simulink library "SMDFR_lib"  (R2024b)
settings: Solver=VariableStepAuto  StartTime=0.0  StopTime=10.0  RelTol=1e-3
undefined symbols (not defined in the file or in its folder): A_cucl, A_cucl2, A_cuocl, A_d, A_fw, A_h, A_h2, A_h20, A_hcl, A_o, A_wc, alfa_c, alfa_f, beta, beta_i, C_cucl, C_cuocl, C_dst, C_h20, C_hcl, C_hst, C_i0, C_o, c_pc, c_pf, c_pw, Ce_i0, d_dst, d_hst, DiscIntNeverNeededParam, E_d, E_e, E_h, E_hte, eta, G_cucl, G_cucl2, G_cuocl, G_h2, G_h20, G_h20i, G_h20o, G_hcl, G_o, h_dpo, h_fw, h_hpo, h_in, h_out, h_wc, k_d, K_d, k_e, k_h, K_h, k_hte, L, Lambda, lambda_c, lambda_e ... (+38)
libraries: simulink x1
settings Model: Creator=ste08  LastModifiedBy=stefanomarchetti
settings RTWCC: GPUComputeCapability=3.5

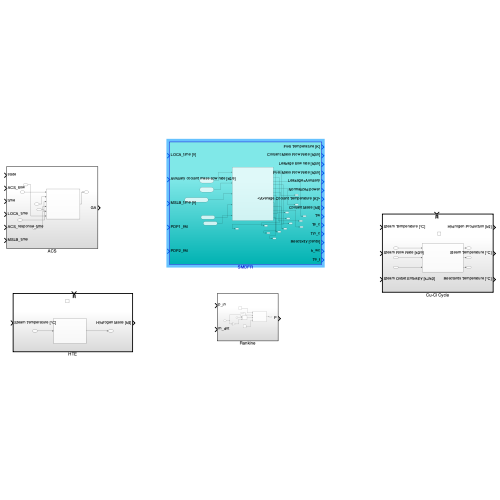
[thumbnail: Simulink's stored preview of the top-level diagram]
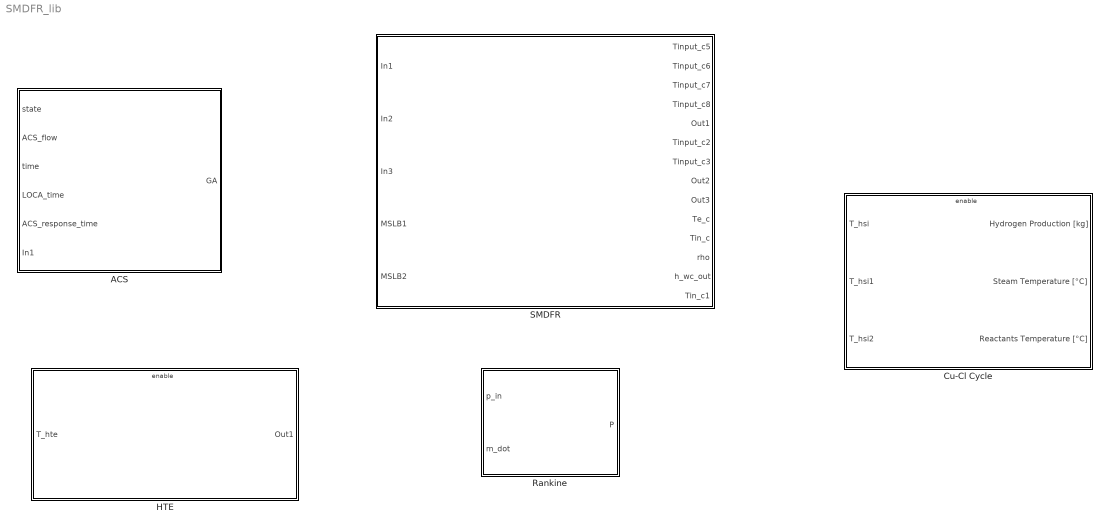
== system SMDFR_lib ==
  ACS : Subsystem
  Cu-Cl Cycle : Subsystem
  HTE : Subsystem
  Rankine : Subsystem
  SMDFR : Subsystem

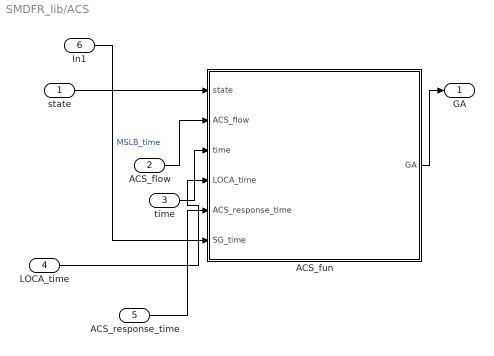
== system SMDFR_lib/ACS ==
  state : Inport
  ACS_flow : Inport  Port=2
  time : Inport  Port=3
  LOCA_time : Inport  Port=4
  ACS_response_time : Inport  Port=5
  In1 : Inport  Port=6
  ACS_fun : MATLAB Function  TreatAsAtomicUnit=on
  GA : Outport
  wires:
  ACS_flow/1 -> ACS_fun/2(ACS_flow)
  state/1 -> ACS_fun/1(state)
  ACS_fun/1(GA) -> GA/1
  time/1 -> ACS_fun/3(time)
  LOCA_time/1 -> ACS_fun/4(LOCA_time)
  ACS_response_time/1 -> ACS_fun/5(ACS_response_time)
  In1/1 -> ACS_fun/6(SG_time)  "MSLB_time"

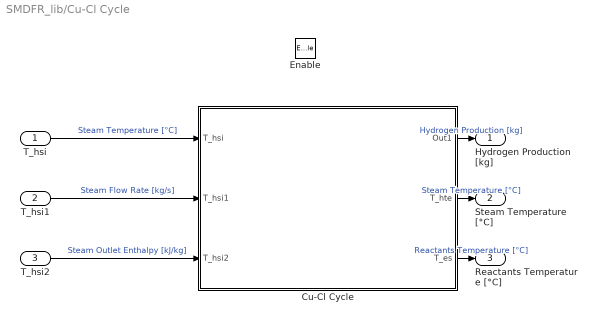
== system SMDFR_lib/Cu-Cl Cycle ==
  T_hsi : Inport
  T_hsi1 : Inport  Port=2
  T_hsi2 : Inport  Port=3
  Enable : EnablePort  StatesWhenEnabling=reset
  Cu-Cl Cycle : Subsystem
  Hydrogen Production [kg] : Outport
  Steam Temperature [°C] : Outport  Port=2
  Reactants Temperature [°C] : Outport  Port=3
  wires:
  Cu-Cl Cycle/1(Out1) -> Hydrogen Production [kg]/1  "Hydrogen Production [kg]"
  T_hsi/1 -> Cu-Cl Cycle/1(T_hsi)  "Steam Temperature [°C]"
  T_hsi1/1 -> Cu-Cl Cycle/2(T_hsi1)  "Steam Flow Rate [kg/s]"
  T_hsi2/1 -> Cu-Cl Cycle/3(T_hsi2)  "Steam Outlet Enthalpy [kJ/kg]"
  Cu-Cl Cycle/3(T_es) -> Reactants Temperature [°C]/1  "Reactants Temperature [°C]"
  Cu-Cl Cycle/2(T_hte) -> Steam Temperature [°C]/1  "Steam Temperature [°C]"

== system SMDFR_lib/HTE ==
  T_hte : Inport
  Enable : EnablePort  StatesWhenEnabling=reset
  HTE : Subsystem
  Out1 : Outport
  wires:
  HTE/1(Out2) -> Out1/1  "Hydrogen Mass [kg]"
  T_hte/1 -> HTE/1(T_hte)  "Steam Temperature [°C]"

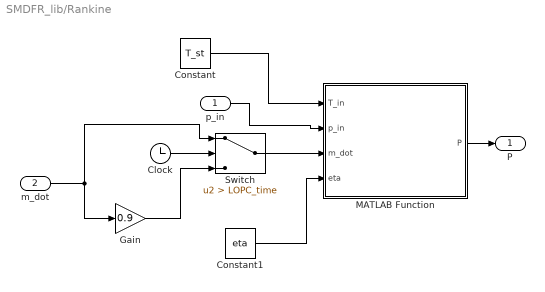
== system SMDFR_lib/Rankine ==
  p_in : Inport
  m_dot : Inport  Port=2
  Clock : Clock
  Constant : Constant  Value=T_st
  Constant1 : Constant  Value=eta
  Gain : Gain  Gain=0.9
  MATLAB Function : MATLAB Function  TreatAsAtomicUnit=on
  Switch : Switch  Criteria=u2 > Threshold  Threshold=LOPC_time  SaturateOnIntegerOverflow=off  InputSameDT=off
  P : Outport
  wires:
  p_in/1 -> MATLAB Function/2(p_in)
  m_dot/1 -> Switch/1, Gain/1
  MATLAB Function/1(P) -> P/1
  Constant/1 -> MATLAB Function/1(T_in)
  Constant1/1 -> MATLAB Function/4(eta)
  Clock/1 -> Switch/2
  Switch/1 -> MATLAB Function/3(m_dot)
  Gain/1 -> Switch/3

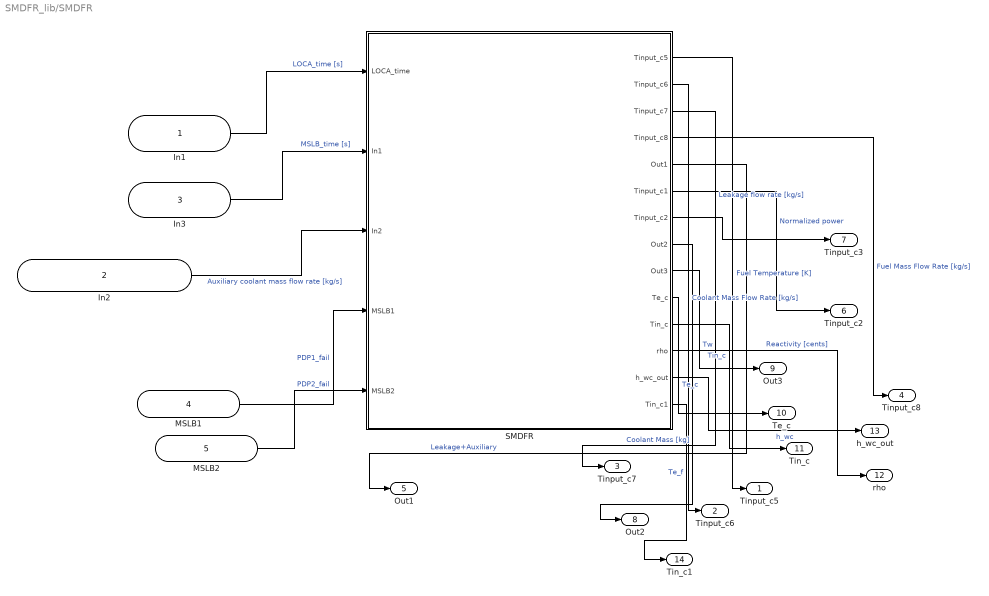
== system SMDFR_lib/SMDFR ==
  In1 : Inport
  In2 : Inport  Port=2
  In3 : Inport  Port=3
  MSLB1 : Inport  Port=4
  MSLB2 : Inport  Port=5
  SMDFR : Subsystem
  Tinput_c5 : Outport
  Tinput_c6 : Outport  Port=2
  Tinput_c7 : Outport  Port=3
  Tinput_c8 : Outport  Port=4
  Out1 : Outport  Port=5
  Tinput_c2 : Outport  Port=6
  Tinput_c3 : Outport  Port=7
  Out2 : Outport  Port=8
  Out3 : Outport  Port=9
  Te_c : Outport  Port=10
  Tin_c : Outport  Port=11
  rho : Outport  Port=12
  h_wc_out : Outport  Port=13
  Tin_c1 : Outport  Port=14
  wires:
  In1/1 -> SMDFR/1(LOCA_time)  "LOCA_time [s]"
  SMDFR/1(Tinput_c5) -> Tinput_c5/1  "Fuel Temperature [K]"
  SMDFR/2(Tinput_c6) -> Tinput_c6/1  "Coolant Mass Flow Rate [kg/s]"
  In2/1 -> SMDFR/3(In2)  "Auxiliary coolant mass flow rate [kg/s]"
  SMDFR/3(Tinput_c7) -> Tinput_c7/1  "Leakage flow rate [kg/s]"
  SMDFR/4(Tinput_c8) -> Tinput_c8/1  "Fuel Mass Flow Rate [kg/s]"
  SMDFR/5(Out1) -> Out1/1  "Leakage+Auxiliary"
  SMDFR/6(Tinput_c1) -> Tinput_c2/1  "Normalized power"
  SMDFR/7(Tinput_c2) -> Tinput_c3/1
  SMDFR/8(Out2) -> Out2/1  "Coolant Mass [kg]"
  SMDFR/9(Out3) -> Out3/1  "Tw"
  SMDFR/10(Te_c) -> Te_c/1  "Te_c"
  SMDFR/11(Tin_c) -> Tin_c/1  "Tin_c"
  SMDFR/12(rho) -> rho/1  "Reactivity [cents]"
  SMDFR/13(h_wc_out) -> h_wc_out/1  "h_wc"
  SMDFR/14(Tin_c1) -> Tin_c1/1  "Te_f"
  In3/1 -> SMDFR/2(In1)  "MSLB_time [s]"
  MSLB1/1 -> SMDFR/4(MSLB1)  "PDP1_fail"
  MSLB2/1 -> SMDFR/5(MSLB2)  "PDP2_fail"

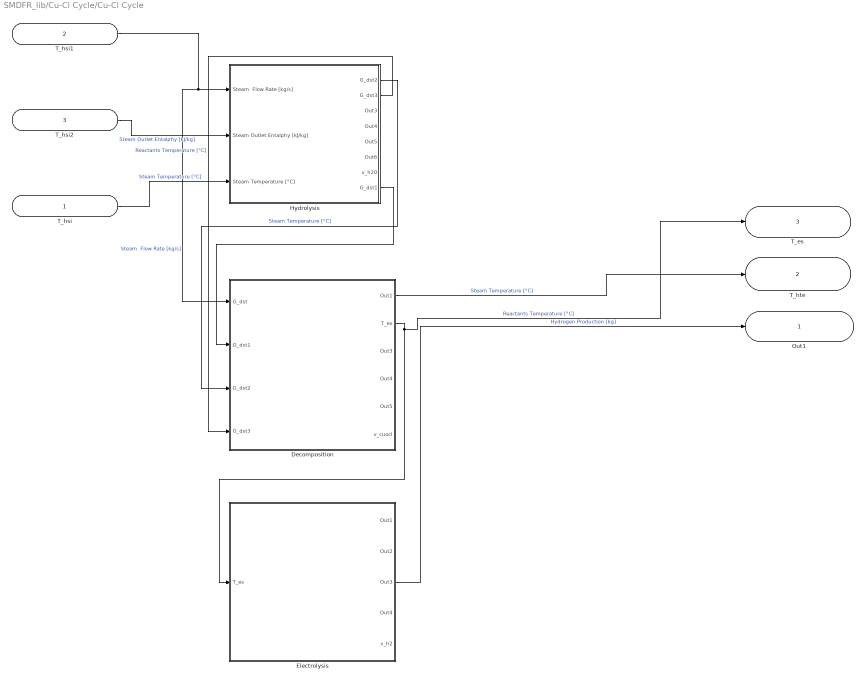
== system SMDFR_lib/Cu-Cl Cycle/Cu-Cl Cycle ==
  T_hsi : Inport
  T_hsi1 : Inport  Port=2
  T_hsi2 : Inport  Port=3
  Decomposition : Subsystem
  Electrolysis : Subsystem
  Hydrolysis : Subsystem
  Out1 : Outport
  T_hte : Outport  Port=2
  T_es : Outport  Port=3
  wires:
  T_hsi2/1 -> Hydrolysis/2(Steam Outlet Entalphy [kJ/kg])  "Steam Outlet Entalphy [kJ/kg]"
  T_hsi/1 -> Hydrolysis/3(Steam Temperature [°C])  "Steam Temperature [°C]"
  Hydrolysis/1(G_dst2) -> Decomposition/3(G_dst2)  "Steam Temperature [°C]"
  Hydrolysis/2(G_dst3) -> Decomposition/4(G_dst3)  "Reactants Temperature [°C]"
  Hydrolysis/8(G_dst1) -> Decomposition/2(G_dst1)
  Decomposition/1(Out1) -> T_hte/1  "Steam Temperature [°C]"
  Decomposition/2(T_es) -> Electrolysis/1(T_es), T_es/1  "Reactants Temperature [°C]"
  Electrolysis/3(Out3) -> Out1/1  "Hydrogen Production [kg]"
  T_hsi1/1 -> Decomposition/1(G_dst), Hydrolysis/1(Steam  Flow Rate [kg/s])  "Steam  Flow Rate [kg/s]"

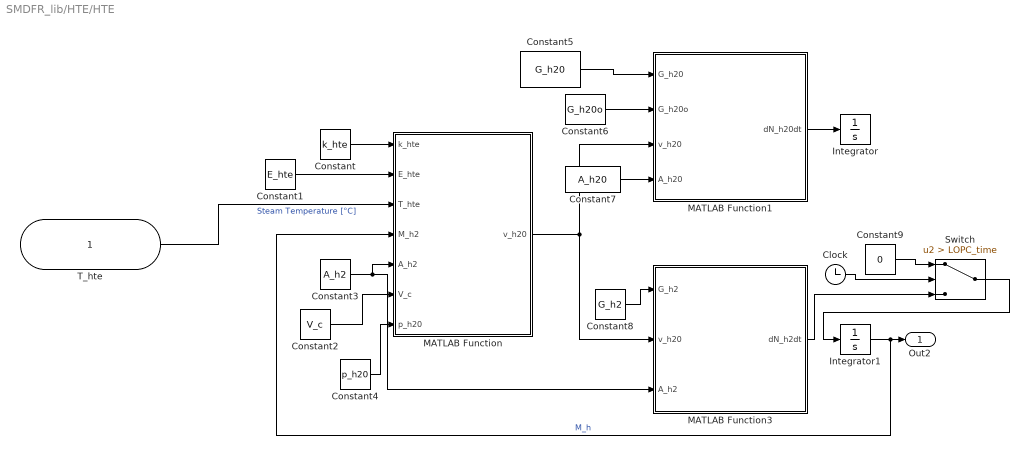
== system SMDFR_lib/HTE/HTE ==
  T_hte : Inport
  Clock : Clock
  Constant : Constant  Value=k_hte
  Constant1 : Constant  Value=E_hte
  Constant2 : Constant  Value=V_c
  Constant3 : Constant  Value=A_h2
  Constant4 : Constant  Value=p_h20
  Constant5 : Constant  Value=G_h20
  Constant6 : Constant  Value=G_h20o
  Constant7 : Constant  Value=A_h20
  Constant8 : Constant  Value=G_h2
  Constant9 : Constant  Value=0
  Integrator : Integrator  InitialCondition=100
  Integrator1 : Integrator  InitialCondition=100
  MATLAB Function : MATLAB Function  TreatAsAtomicUnit=on
  MATLAB Function1 : MATLAB Function  TreatAsAtomicUnit=on
  MATLAB Function3 : MATLAB Function  TreatAsAtomicUnit=on
  Switch : Switch  Criteria=u2 > Threshold  Threshold=LOPC_time  SaturateOnIntegerOverflow=off  InputSameDT=off
  Out2 : Outport
  wires:
  T_hte/1 -> MATLAB Function/3(T_hte)  "Steam Temperature [°C]"
  MATLAB Function/1(v_h20) -> MATLAB Function3/2(v_h20), MATLAB Function1/3(v_h20)
  Constant/1 -> MATLAB Function/1(k_hte)
  Constant1/1 -> MATLAB Function/2(E_hte)
  Constant3/1 -> MATLAB Function3/3(A_h2), MATLAB Function/5(A_h2)
  Constant2/1 -> MATLAB Function/6(V_c)
  Constant4/1 -> MATLAB Function/7(p_h20)
  Constant5/1 -> MATLAB Function1/1(G_h20)
  Constant6/1 -> MATLAB Function1/2(G_h20o)
  Constant7/1 -> MATLAB Function1/4(A_h20)
  Constant8/1 -> MATLAB Function3/1(G_h2)
  MATLAB Function1/1(dN_h20dt) -> Integrator/1
  Switch/1 -> Integrator1/1
  Integrator1/1 -> MATLAB Function/4(M_h2), Out2/1  "M_h"
  MATLAB Function3/1(dN_h2dt) -> Switch/3
  Constant9/1 -> Switch/1
  Clock/1 -> Switch/2

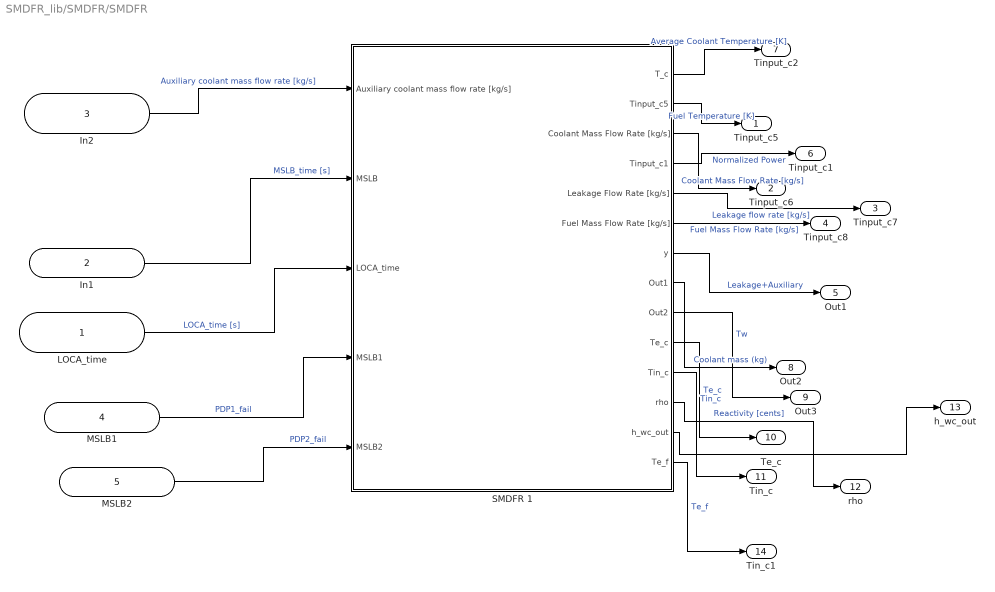
== system SMDFR_lib/SMDFR/SMDFR ==
  LOCA_time : Inport
  In1 : Inport  Port=2
  In2 : Inport  Port=3
  MSLB1 : Inport  Port=4
  MSLB2 : Inport  Port=5
  SMDFR 1 : Subsystem
  Tinput_c5 : Outport
  Tinput_c6 : Outport  Port=2
  Tinput_c7 : Outport  Port=3
  Tinput_c8 : Outport  Port=4
  Out1 : Outport  Port=5
  Tinput_c1 : Outport  Port=6
  Tinput_c2 : Outport  Port=7
  Out2 : Outport  Port=8
  Out3 : Outport  Port=9
  Te_c : Outport  Port=10
  Tin_c : Outport  Port=11
  rho : Outport  Port=12
  h_wc_out : Outport  Port=13
  Tin_c1 : Outport  Port=14
  wires:
  SMDFR 1/3(Coolant Mass Flow Rate [kg/s]) -> Tinput_c6/1  "Coolant Mass Flow Rate [kg/s]"
  SMDFR 1/2(Tinput_c5) -> Tinput_c5/1  "Fuel Temperature [K]"
  In2/1 -> SMDFR 1/1(Auxiliary coolant mass flow rate [kg/s])  "Auxiliary coolant mass flow rate [kg/s]"
  SMDFR 1/5(Leakage Flow Rate [kg/s]) -> Tinput_c7/1  "Leakage flow rate [kg/s]"
  SMDFR 1/6(Fuel Mass Flow Rate [kg/s]) -> Tinput_c8/1  "Fuel Mass Flow Rate [kg/s]"
  LOCA_time/1 -> SMDFR 1/3(LOCA_time)  "LOCA_time [s]"
  SMDFR 1/7(y) -> Out1/1  "Leakage+Auxiliary"
  SMDFR 1/4(Tinput_c1) -> Tinput_c1/1  "Normalized Power"
  SMDFR 1/1(T_c) -> Tinput_c2/1  "Average Coolant Temperature [K]"
  SMDFR 1/8(Out1) -> Out2/1  "Coolant mass (kg)"
  SMDFR 1/9(Out2) -> Out3/1  "Tw"
  SMDFR 1/10(Te_c) -> Te_c/1  "Te_c"
  SMDFR 1/11(Tin_c) -> Tin_c/1  "Tin_c"
  SMDFR 1/12(rho) -> rho/1  "Reactivity [cents]"
  SMDFR 1/13(h_wc_out) -> h_wc_out/1
  SMDFR 1/14(Te_f) -> Tin_c1/1  "Te_f"
  In1/1 -> SMDFR 1/2(MSLB)  "MSLB_time [s]"
  MSLB1/1 -> SMDFR 1/4(MSLB1)  "PDP1_fail"
  MSLB2/1 -> SMDFR 1/5(MSLB2)  "PDP2_fail"

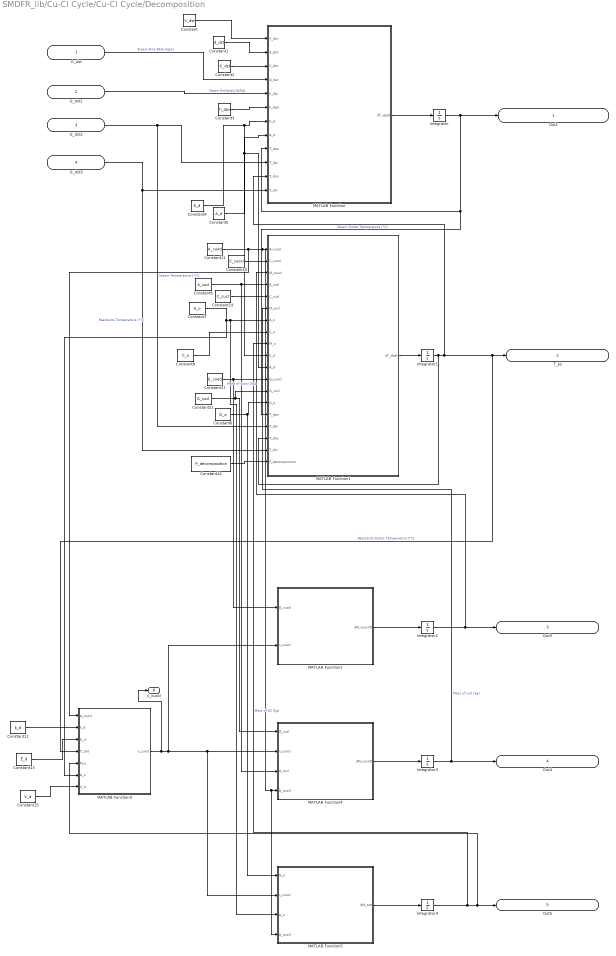
== system SMDFR_lib/Cu-Cl Cycle/Cu-Cl Cycle/Decomposition ==
  G_dst : Inport
  G_dst1 : Inport  Port=2
  G_dst2 : Inport  Port=3
  G_dst3 : Inport  Port=4
  Constant : Constant  Value=V_dst
  Constant1 : Constant  Value=d_dst
  Constant10 : Constant  Value=C_cuocl
  Constant11 : Constant  Value=A_cuocl
  Constant12 : Constant  Value=k_d
  Constant13 : Constant  Value=E_d
  Constant14 : Constant  Value=P_decomposition
  Constant15 : Constant  Value=V_d
  Constant17 : Constant  Value=G_cuocl
  Constant19 : Constant  Value=C_cucl
  Constant2 : Constant  Value=C_dst
  Constant21 : Constant  Value=G_cucl
  Constant3 : Constant  Value=h_dpo
  Constant4 : Constant  Value=K_d
  Constant5 : Constant  Value=A_d
  Constant6 : Constant  Value=G_o
  Constant7 : Constant  Value=A_o
  Constant8 : Constant  Value=C_o
  Constant9 : Constant  Value=A_cucl
  Integrator : Integrator  InitialCondition=1000
  Integrator{1..4} (4 alike) : Integrator  InitialCondition=100
  MATLAB Function : MATLAB Function  TreatAsAtomicUnit=on
  MATLAB Function1 : MATLAB Function  TreatAsAtomicUnit=on
  MATLAB Function2 : MATLAB Function  TreatAsAtomicUnit=on
  MATLAB Function3 : MATLAB Function  TreatAsAtomicUnit=on
  MATLAB Function4 : MATLAB Function  TreatAsAtomicUnit=on
  MATLAB Function5 : MATLAB Function  TreatAsAtomicUnit=on
  Out1 : Outport
  T_es : Outport  Port=2
  Out3 : Outport  Port=3
  Out4 : Outport  Port=4
  Out5 : Outport  Port=5
  v_cuocl : Outport  Port=6
  wires:
  MATLAB Function/1(dT_dpdt) -> Integrator/1
  G_dst/1 -> MATLAB Function/4(G_dst)  "Steam Flow Rate [kg/s]"
  G_dst1/1 -> MATLAB Function/5(h_dpi)  "Steam Enthalpy [kJ/kg]"
  G_dst2/1 -> MATLAB Function1/16(T_dpi), MATLAB Function/10(T_dpi)  "Steam Temperature [°C]"
  Constant/1 -> MATLAB Function/1(V_dst)
  Constant1/1 -> MATLAB Function/2(d_dst)
  Constant2/1 -> MATLAB Function/3(C_dst)
  Constant3/1 -> MATLAB Function/6(h_dpo)
  Constant4/1 -> MATLAB Function/7(K_d), MATLAB Function1/10(K_d)
  Constant5/1 -> MATLAB Function/8(A_d), MATLAB Function1/11(A_d)
  G_dst3/1 -> MATLAB Function1/18(T_dsi), MATLAB Function/12(T_dsi)  "Reactants Temperature [°C]"
  MATLAB Function1/1(dT_dsdt) -> Integrator1/1
  Integrator/1 -> MATLAB Function1/15(T_dpo), MATLAB Function/9(T_dpo), Out1/1  "Steam Outlet Temperature [°C]"
  Integrator1/1 -> MATLAB Function1/17(T_dso), MATLAB Function/11(T_dso), MATLAB Function3/4(T_dso), T_es/1  "Reactants Outlet Temperature [°C]"
  Constant11/1 -> MATLAB Function5/4(A_cuocl), MATLAB Function4/4(A_cuocl), MATLAB Function1/1(A_cuocl), MATLAB Function3/1(A_cuocl)
  Constant9/1 -> MATLAB Function4/3(A_cucl), MATLAB Function1/4(A_cucl)
  Constant21/1 -> MATLAB Function4/1(G_cucl), MATLAB Function1/13(G_cucl)
  Constant17/1 -> MATLAB Function2/1(G_cuocl), MATLAB Function1/12(G_cuocl)
  Constant6/1 -> MATLAB Function5/1(G_o), MATLAB Function1/14(G_o)
  Constant7/1 -> MATLAB Function3/6(A_o), MATLAB Function5/3(A_o), MATLAB Function1/7(A_o)
  Constant8/1 -> MATLAB Function1/8(C_o)
  Constant10/1 -> MATLAB Function1/2(C_cuocl)
  Constant19/1 -> MATLAB Function1/5(C_cucl)
  Constant14/1 -> MATLAB Function1/19(P_decomposition)
  MATLAB Function2/1(dM_cuocldt) -> Integrator2/1
  Integrator2/1 -> MATLAB Function1/3(M_cuocl), Out3/1  "Mass of cuocl [kg]"
  MATLAB Function3/1(v_cuocl) -> v_cuocl/1, MATLAB Function2/2(v_cuocl), MATLAB Function5/2(v_cuocl), MATLAB Function4/2(v_cuocl)
  MATLAB Function4/1(dM_cucldt) -> Integrator3/1
  Integrator3/1 -> MATLAB Function1/6(M_cucl), Out4/1  "Mass of cucl [kg]"
  MATLAB Function5/1(dM_odt) -> Integrator4/1
  Integrator4/1 -> MATLAB Function1/9(M_o), MATLAB Function3/5(M_o), Out5/1  "Mass of O2 [kg]"
  Constant15/1 -> MATLAB Function3/7(V_d)
  Constant13/1 -> MATLAB Function3/3(E_d)
  Constant12/1 -> MATLAB Function3/2(k_d)

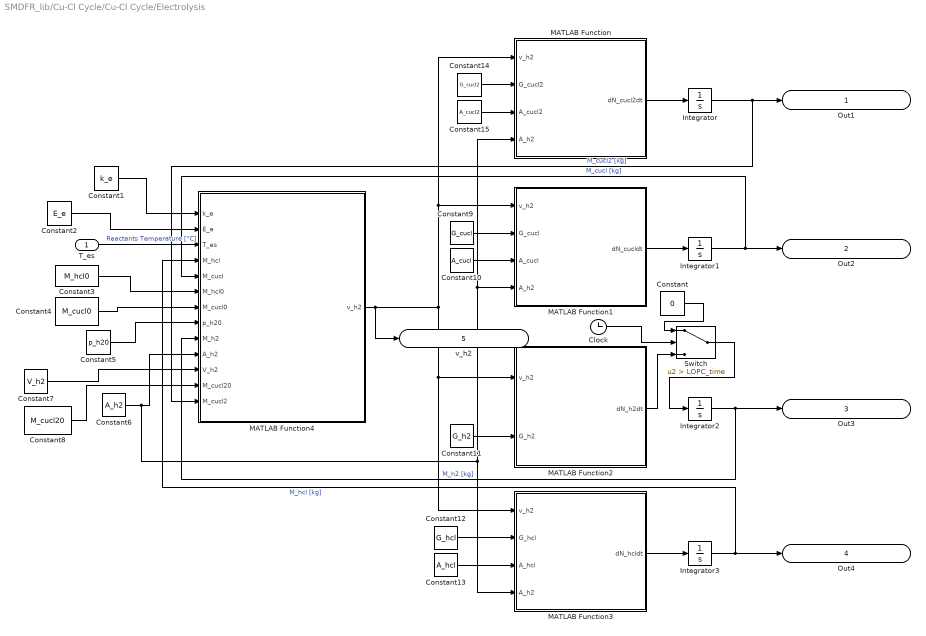
== system SMDFR_lib/Cu-Cl Cycle/Cu-Cl Cycle/Electrolysis ==
  T_es : Inport
  Clock : Clock
  Constant : Constant  Value=0
  Constant1 : Constant  Value=k_e
  Constant10 : Constant  Value=A_cucl
  Constant11 : Constant  Value=G_h2
  Constant12 : Constant  Value=G_hcl
  Constant13 : Constant  Value=A_hcl
  Constant14 : Constant  Value=G_cucl2
  Constant15 : Constant  Value=A_cucl2
  Constant2 : Constant  Value=E_e
  Constant3 : Constant  Value=M_hcl0
  Constant4 : Constant  Value=M_cucl0
  Constant5 : Constant  Value=p_h20
  Constant6 : Constant  Value=A_h2
  Constant7 : Constant  Value=V_h2
  Constant8 : Constant  Value=M_cucl20
  Constant9 : Constant  Value=G_cucl
  Integrator : Integrator  InitialCondition=M_cucl20
  Integrator1 : Integrator  InitialCondition=M_cucl0
  Integrator2 : Integrator  InitialCondition=M_h20
  Integrator3 : Integrator  InitialCondition=M_hcl0
  MATLAB Function : MATLAB Function  TreatAsAtomicUnit=on
  MATLAB Function1 : MATLAB Function  TreatAsAtomicUnit=on
  MATLAB Function2 : MATLAB Function  TreatAsAtomicUnit=on
  MATLAB Function3 : MATLAB Function  TreatAsAtomicUnit=on
  MATLAB Function4 : MATLAB Function  TreatAsAtomicUnit=on
  Switch : Switch  Criteria=u2 > Threshold  Threshold=LOPC_time  SaturateOnIntegerOverflow=off  InputSameDT=off
  Out1 : Outport
  Out2 : Outport  Port=2
  Out3 : Outport  Port=3
  Out4 : Outport  Port=4
  v_h2 : Outport  Port=5
  wires:
  MATLAB Function/1(dN_cucl2dt) -> Integrator/1
  MATLAB Function1/1(dN_cucldt) -> Integrator1/1
  Switch/1 -> Integrator2/1
  MATLAB Function3/1(dN_hcldt) -> Integrator3/1
  MATLAB Function4/1(v_h2) -> v_h2/1, MATLAB Function/1(v_h2), MATLAB Function1/1(v_h2), MATLAB Function3/1(v_h2), MATLAB Function2/1(v_h2)
  Integrator/1 -> MATLAB Function4/13(M_cucl2), Out1/1  "M_cucl2 [kg]"
  Integrator1/1 -> MATLAB Function4/5(M_cucl), Out2/1  "M_cucl [kg]"
  Integrator2/1 -> MATLAB Function4/9(M_h2), Out3/1  "M_h2 [kg]"
  Integrator3/1 -> MATLAB Function4/4(M_hcl), Out4/1  "M_hcl [kg]"
  T_es/1 -> MATLAB Function4/3(T_es)  "Reactants Temperature [°C]"
  Constant1/1 -> MATLAB Function4/1(k_e)
  Constant2/1 -> MATLAB Function4/2(E_e)
  Constant3/1 -> MATLAB Function4/6(M_hcl0)
  Constant4/1 -> MATLAB Function4/7(M_cucl0)
  Constant5/1 -> MATLAB Function4/8(p_h20)
  Constant6/1 -> MATLAB Function/4(A_h2), MATLAB Function1/4(A_h2), MATLAB Function3/4(A_h2), MATLAB Function4/10(A_h2)
  Constant7/1 -> MATLAB Function4/11(V_h2)
  Constant8/1 -> MATLAB Function4/12(M_cucl20)
  Constant9/1 -> MATLAB Function1/2(G_cucl)
  Constant10/1 -> MATLAB Function1/3(A_cucl)
  Constant11/1 -> MATLAB Function2/2(G_h2)
  Constant12/1 -> MATLAB Function3/2(G_hcl)
  Constant13/1 -> MATLAB Function3/3(A_hcl)
  Constant14/1 -> MATLAB Function/2(G_cucl2)
  Constant15/1 -> MATLAB Function/3(A_cucl2)
  MATLAB Function2/1(dN_h2dt) -> Switch/3
  Clock/1 -> Switch/2
  Constant/1 -> Switch/1

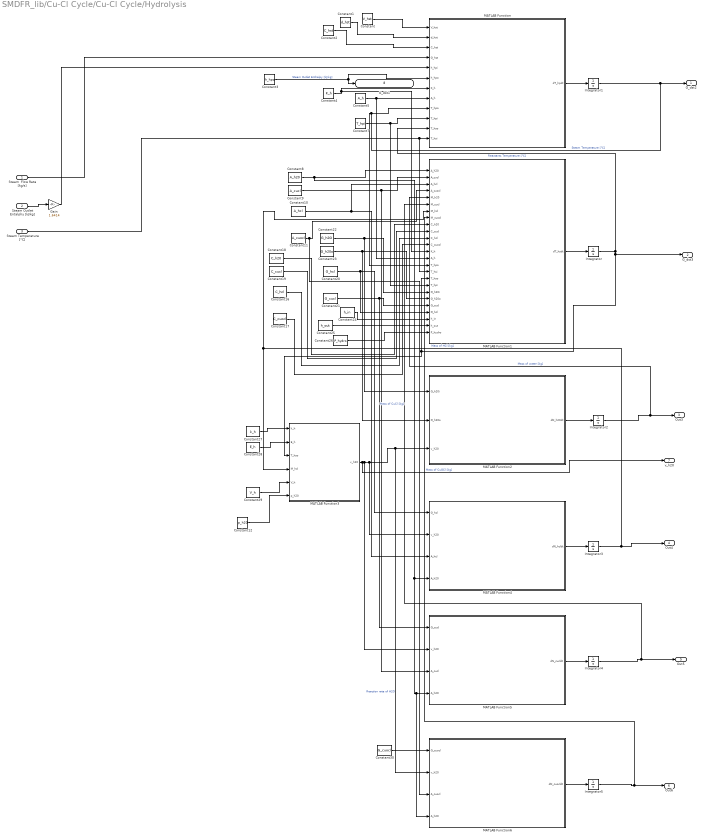
== system SMDFR_lib/Cu-Cl Cycle/Cu-Cl Cycle/Hydrolysis ==
  Steam  Flow Rate [kg/s] : Inport
  Steam Outlet Entalphy [kJ/kg] : Inport  Port=2
  Steam Temperature [°C] : Inport  Port=3
  Constant : Constant  Value=V_hst
  Constant1 : Constant  Value=d_hst
  Constant10 : Constant  Value=A_hcl
  Constant11 : Constant  Value=A_cuocl
  Constant12 : Constant  Value=p_h20
  Constant16 : Constant  Value=C_hcl
  Constant17 : Constant  Value=C_cuocl
  Constant18 : Constant  Value=C_h20
  Constant19 : Constant  Value=C_cucl
  Constant2 : Constant  Value=C_hst
  Constant20 : Constant  Value=G_hcl
  Constant21 : Constant  Value=G_cucl
  Constant22 : Constant  Value=G_h20i
  Constant23 : Constant  Value=G_h20o
  Constant24 : Constant  Value=h_in
  Constant25 : Constant  Value=h_out
  Constant26 : Constant  Value=P_hydro
  Constant27 : Constant  Value=k_h
  Constant28 : Constant  Value=E_h
  Constant29 : Constant  Value=V_h
  Constant3 : Constant  Value=h_hpo
  Constant30 : Constant  Value=G_cuocl
  Constant4 : Constant  Value=K_h
  Constant5 : Constant  Value=A_h
  Constant7 : Constant  Value=T_hpi
  Constant8 : Constant  Value=A_h20
  Constant9 : Constant  Value=A_cucl
  Gain : Gain  Gain=1.6414
  Integrator : Integrator  InitialCondition=T_hpi-50
  Integrator1 : Integrator  InitialCondition=T_st+100
  Integrator2 : Integrator  InitialCondition=200
  Integrator3 : Integrator  InitialCondition=50
  Integrator4 : Integrator  InitialCondition=200
  Integrator5 : Integrator  InitialCondition=50
  MATLAB Function : MATLAB Function  TreatAsAtomicUnit=on
  MATLAB Function1 : MATLAB Function  TreatAsAtomicUnit=on
  MATLAB Function2 : MATLAB Function  TreatAsAtomicUnit=on
  MATLAB Function3 : MATLAB Function  TreatAsAtomicUnit=on
  MATLAB Function4 : MATLAB Function  TreatAsAtomicUnit=on
  MATLAB Function5 : MATLAB Function  TreatAsAtomicUnit=on
  MATLAB Function6 : MATLAB Function  TreatAsAtomicUnit=on
  G_dst2 : Outport
  G_dst3 : Outport  Port=2
  Out3 : Outport  Port=3
  Out4 : Outport  Port=4
  Out5 : Outport  Port=5
  Out6 : Outport  Port=6
  v_h20 : Outport  Port=7
  G_dst1 : Outport  Port=8
  wires:
  Constant23/1 -> MATLAB Function2/2(G_h20o), MATLAB Function1/20(G_h20o)
  MATLAB Function3/1(v_h20) -> v_h20/1, MATLAB Function5/2(v_h20), MATLAB Function4/2(v_h20), MATLAB Function6/2(v_h20), MATLAB Function2/3(v_h20)  "Reaction rate of H2O"
  Constant8/1 -> MATLAB Function6/4(A_h20), MATLAB Function5/4(A_h20), MATLAB Function4/4(A_h20), MATLAB Function1/1(A_h20)
  Integrator2/1 -> MATLAB Function1/5(M_h20), Out3/1  "Mass of water [kg]"
  Constant26/1 -> MATLAB Function1/25(P_hydro)
  Constant/1 -> MATLAB Function/1(V_hst)
  Integrator4/1 -> MATLAB Function1/6(M_cucl), Out5/1  "Mass of CuCl [kg]"
  Constant27/1 -> MATLAB Function3/1(k_h)
  Integrator/1 -> G_dst3/1, MATLAB Function3/3(T_hso), MATLAB Function1/17(T_hso), MATLAB Function/11(T_hso)  "Reactants Temperature [°C]"
  Constant25/1 -> MATLAB Function1/24(h_out)
  Steam Temperature [°C]/1 -> MATLAB Function1/16(T_hsi), MATLAB Function/12(T_hsi)
  Constant28/1 -> MATLAB Function3/2(E_h)
  Constant24/1 -> MATLAB Function1/23(h_in)
  Constant3/1 -> G_dst1/1, MATLAB Function/6(h_hpo)  "Steam Outlet Enthalpy [kJ/kg]"
  Constant1/1 -> MATLAB Function/2(d_hst)
  Integrator1/1 -> MATLAB Function1/15(T_hpo), MATLAB Function/9(T_hpo), G_dst2/1  "Steam Temperature [°C]"
  Constant20/1 -> MATLAB Function4/1(G_hcl), MATLAB Function1/22(G_hcl)
  Constant7/1 -> MATLAB Function1/18(T_hpi), MATLAB Function/10(T_hpi)
  Constant2/1 -> MATLAB Function/3(C_hst)
  Gain/1 -> MATLAB Function/5(h_hpi)
  Constant22/1 -> MATLAB Function2/1(G_h20i), MATLAB Function1/19(G_h20i)
  Constant9/1 -> MATLAB Function5/3(A_cucl), MATLAB Function1/2(A_cucl)
  Constant21/1 -> MATLAB Function5/1(G_cucl), MATLAB Function1/21(G_cucl)
  Constant4/1 -> MATLAB Function1/13(K_h), MATLAB Function/7(K_h)
  Constant11/1 -> MATLAB Function6/3(A_cuocl), MATLAB Function1/4(A_cuocl)
  Constant19/1 -> MATLAB Function1/10(C_cucl)
  Integrator5/1 -> MATLAB Function1/8(M_cuocl), Out6/1  "Mass of CuOCl [kg]"
  MATLAB Function4/1(dN_hcldt) -> Integrator3/1
  Constant29/1 -> MATLAB Function3/5(V_h)
  Constant16/1 -> MATLAB Function1/11(C_hcl)
  MATLAB Function6/1(dN_cuocldt) -> Integrator5/1
  Constant17/1 -> MATLAB Function1/12(C_cuocl)
  Constant10/1 -> MATLAB Function4/3(A_hcl), MATLAB Function1/3(A_hcl)
  MATLAB Function5/1(dN_cucldt) -> Integrator4/1
  MATLAB Function/1(dT_hpdt) -> Integrator1/1
  Constant5/1 -> MATLAB Function1/14(A_h), MATLAB Function/8(A_h)
  Constant30/1 -> MATLAB Function6/1(G_cuocl)
  MATLAB Function1/1(dT_hsdt) -> Integrator/1
  Constant18/1 -> MATLAB Function1/9(C_h20)
  Integrator3/1 -> Out4/1, MATLAB Function1/7(M_hcl), MATLAB Function3/4(M_hcl)  "Mass of HCl [kg]"
  MATLAB Function2/1(dN_h20dt) -> Integrator2/1
  Steam  Flow Rate [kg/s]/1 -> MATLAB Function/4(G_hst)
  Constant12/1 -> MATLAB Function3/6(p_h20)
  Steam Outlet Entalphy [kJ/kg]/1 -> Gain/1

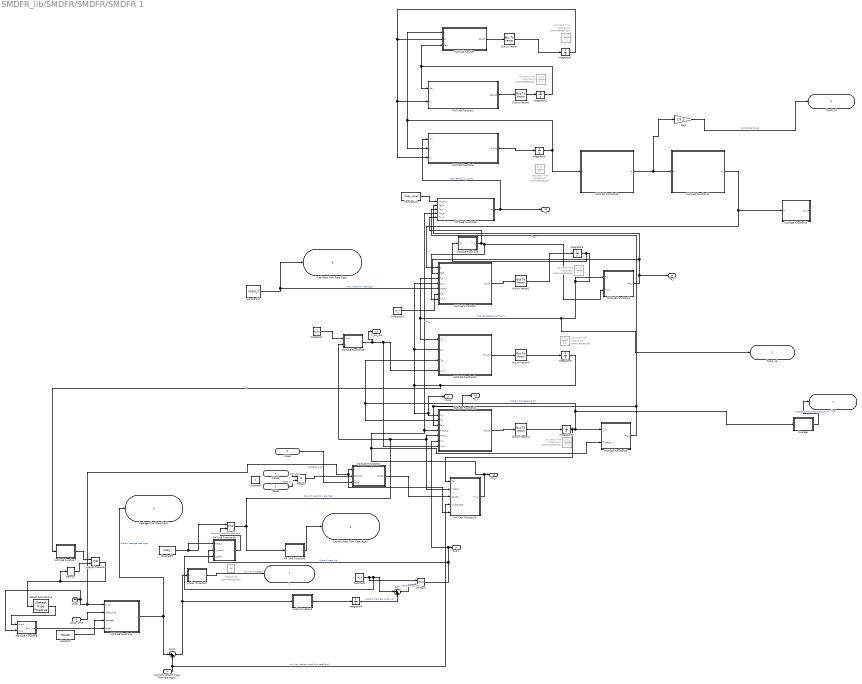
== system SMDFR_lib/SMDFR/SMDFR/SMDFR 1 ==
  Auxiliary coolant mass flow rate [kg/s] : Inport
  MSLB : Inport  Port=2
  LOCA_time : Inport  Port=3
  MSLB1 : Inport  Port=4
  MSLB2 : Inport  Port=5
  Average : MATLAB Function  TreatAsAtomicUnit=on
  Bus to Vector{,1..4} (5 alike) : BusToVector
  Clock : Clock
  Constant : Constant  Value=leakage
  Constant1 : Constant  Value=M_c
  Constant13 : Constant  Value=rhoex_value  SampleTime=-1
  Constant17 : Constant  Value=mdot_f  SampleTime=-1
  Constant2 : Constant  Value=h_wc
  Constant20 : Constant  Value=M_f  SampleTime=-1
  Constant3 : Constant
  Constant9 : Constant  Value=mdot_c  SampleTime=-1
  Detect Rise Positive : simulink/Logic and Bit Operations/Detect Rise Positive  vinit=0  OutDataTypeStr=boolean
  Discrete-Time Integrator : DiscreteIntegrator  Commented=on  InitialCondition=Tf_0  SampleTime=-1  ICPrevOutput=DiscIntNeverNeededParam  ICPrevScaledInput=DiscIntNeverNeededParam
  Discrete-Time Integrator2 : DiscreteIntegrator  Commented=on  InitialCondition=N_0  SampleTime=-1  ICPrevOutput=DiscIntNeverNeededParam  ICPrevScaledInput=DiscIntNeverNeededParam
  Discrete-Time Integrator3 : DiscreteIntegrator  Commented=on  InitialCondition=Ce_i0  SampleTime=-1  ICPrevOutput=DiscIntNeverNeededParam  ICPrevScaledInput=DiscIntNeverNeededParam
  Discrete-Time Integrator4 : DiscreteIntegrator  Commented=on  InitialCondition=C_i0  SampleTime=-1  ICPrevOutput=DiscIntNeverNeededParam  ICPrevScaledInput=DiscIntNeverNeededParam
  Discrete-Time Integrator5 : DiscreteIntegrator  Commented=on  InitialCondition=Tw_0  SampleTime=-1  ICPrevOutput=DiscIntNeverNeededParam  ICPrevScaledInput=DiscIntNeverNeededParam
  Discrete-Time Integrator6 : DiscreteIntegrator  Commented=on  InitialCondition=Tc_0  SampleTime=-1  ICPrevOutput=DiscIntNeverNeededParam  ICPrevScaledInput=DiscIntNeverNeededParam
  Gain : Gain  Gain=1/P_0
  Integrator1 : Integrator  InitialCondition=C_i0
  Integrator10 : Integrator  InitialCondition=Tc_in*ones(3,1)
  Integrator2 : Integrator  InitialCondition=Ce_i0
  Integrator3 : Integrator  InitialCondition=N_0
  Integrator4 : Integrator
  Integrator5 : Integrator  Commented=on
  Integrator8 : Integrator  InitialCondition=Tin_f*ones(3,1)
  Integrator9 : Integrator  InitialCondition=1100*ones(3,1)
  Logical Operator : Logic  Operator=OR  AllPortsSameDT=off  OutDataTypeStr=boolean
  MATLAB Function : MATLAB Function  TreatAsAtomicUnit=on
  MATLAB Function1 : MATLAB Function  TreatAsAtomicUnit=on
  MATLAB Function10 : MATLAB Function  TreatAsAtomicUnit=on
  MATLAB Function11 : MATLAB Function  TreatAsAtomicUnit=on
  MATLAB Function12 : MATLAB Function  TreatAsAtomicUnit=on
  MATLAB Function13 : MATLAB Function  TreatAsAtomicUnit=on
  MATLAB Function14 : MATLAB Function  TreatAsAtomicUnit=on
  MATLAB Function15 : MATLAB Function  TreatAsAtomicUnit=on
  MATLAB Function16 : MATLAB Function  TreatAsAtomicUnit=on
  MATLAB Function17 : MATLAB Function  TreatAsAtomicUnit=on
  MATLAB Function18 : MATLAB Function  TreatAsAtomicUnit=on
  MATLAB Function19 : MATLAB Function  TreatAsAtomicUnit=on
  MATLAB Function2 : MATLAB Function  TreatAsAtomicUnit=on
  MATLAB Function20 : MATLAB Function  TreatAsAtomicUnit=on
  MATLAB Function3 : MATLAB Function  TreatAsAtomicUnit=on
  MATLAB Function4 : MATLAB Function  TreatAsAtomicUnit=on
  MATLAB Function5 : MATLAB Function  TreatAsAtomicUnit=on
  MATLAB Function6 : MATLAB Function  TreatAsAtomicUnit=on
  MATLAB Function7 : MATLAB Function  TreatAsAtomicUnit=on
  MATLAB Function8 : MATLAB Function  TreatAsAtomicUnit=on
  MATLAB Function9 : MATLAB Function  TreatAsAtomicUnit=on
  Memory : Memory
  MinMax : MinMax  Inputs=2
  MinMax1 : MinMax  Inputs=2
  Product : Product
  Sum : Sum  Inputs=|++
  Sum1 : Sum  Inputs=|++
  scalar to vector2 : MATLAB Function  TreatAsAtomicUnit=on
  scalar to vector3 : MATLAB Function  TreatAsAtomicUnit=on
  T_c : Outport
  Tinput_c5 : Outport  Port=2
  Coolant Mass Flow Rate [kg/s] : Outport  Port=3
  Tinput_c1 : Outport  Port=4
  Leakage Flow Rate [kg/s] : Outport  Port=5
  Fuel Mass Flow Rate [kg/s] : Outport  Port=6
  y : Outport  Port=7
  Out1 : Outport  Port=8
  Out2 : Outport  Port=9
  Te_c : Outport  Port=10
  Tin_c : Outport  Port=11
  rho : Outport  Port=12
  h_wc_out : Outport  Port=13
  Te_f : Outport  Port=14
  wires:
  MATLAB Function4/1(y) -> Sum1/1, Leakage Flow Rate [kg/s]/1  "Coolant leakage rate (kg/s)"
  Constant20/1 -> MATLAB Function5/6(M_f)
  Bus to Vector/1 -> Integrator1/1
  Constant13/1 -> MATLAB Function3/1(rho_ext)
  Integrator9/1 -> MATLAB Function7/1(u), Out2/1, MATLAB Function12/1(T_w), MATLAB Function5/4(T_w), MATLAB Function11/2(T_w)  "Tw"
  MinMax/1 -> MATLAB Function6/1(u), MATLAB Function19/2(mdot_c), MATLAB Function10/2(mdot_c), MATLAB Function12/5(mdot_c)  "Coolant mass flow rate (kg/s)"
  Sum1/1 -> scalar to vector2/1(u), scalar to vector3/1(u)
  scalar to vector2/1(y) -> y/1  "Auxiliary+leakage"
  MATLAB Function15/1(Te_c) -> MATLAB Function3/3(Te_c), MATLAB Function12/3(Te_c), Te_c/1  "Te_c"
  MATLAB Function16/1(Te_f) -> MATLAB Function5/2(Te_f), MATLAB Function3/2(Te_f), Te_f/1
  Constant17/1 -> Fuel Mass Flow Rate [kg/s]/1, MATLAB Function5/5(mdot_f)  "Fuel mass flow rate (kg/s)"
  Bus to Vector4/1 -> Integrator10/1
  Gain/1 -> Tinput_c1/1  "Normalized Power"
  MATLAB Function11/1(dT_wdt) -> Bus to Vector3/1
  MATLAB Function/1(dC_idt) -> Bus to Vector/1
  MATLAB Function3/1(rho) -> MATLAB Function2/1(rho), rho/1  "Total Reactivity (cents)"
  Constant9/1 -> MinMax/1, MATLAB Function18/1(mdot_c)
  Integrator2/1 -> MATLAB Function/3(Ce_i), MATLAB Function1/1(Ce_i)
  MATLAB Function12/1(dT_cdt) -> Bus to Vector4/1
  MATLAB Function13/1(P) -> Gain/1, MATLAB Function14/1(P)
  MATLAB Function14/1(Pi) -> MATLAB Function5/1(Pi), MATLAB Function17/1(Pi)
  MATLAB Function5/1(dT_fdt) -> Bus to Vector2/1
  Bus to Vector2/1 -> Integrator8/1
  Bus to Vector1/1 -> Integrator2/1
  MATLAB Function1/1(dCei_dt) -> Bus to Vector1/1
  Integrator1/1 -> MATLAB Function2/3(C_i), MATLAB Function1/2(C_i), MATLAB Function/2(C_i)
  MATLAB Function2/1(dN_dt) -> Integrator3/1
  Integrator3/1 -> MATLAB Function13/1(N), MATLAB Function/1(N), MATLAB Function2/2(N)
  Bus to Vector3/1 -> Integrator9/1
  Average/1(y) -> T_c/1  "Average Coolant Temperature [K]"
  Integrator10/1 -> MATLAB Function10/1(Tc), Average/1(u), MATLAB Function12/2(T_c), MATLAB Function11/3(T_c), MATLAB Function15/1(T_c)  "Coolant Temperature [K]"
  Integrator8/1 -> MATLAB Function9/1(Tf), Tinput_c5/1, MATLAB Function11/1(T_f), MATLAB Function5/3(T_f), MATLAB Function16/1(T_f)  "Fuel temperature profile (K)"
  MATLAB Function6/1(y) -> Coolant Mass Flow Rate [kg/s]/1
  Auxiliary coolant mass flow rate [kg/s]/1 -> MATLAB Function10/4(m_dot_ACS), Sum1/2  "Auxiliary coolant mass flow rate [kg/s]"
  MATLAB Function18/1(y) -> MinMax/2  "Coolant mass flow rate (kg/s)"
  LOCA_time/1 -> MATLAB Function4/2(LOCA_time)
  Constant/1 -> MATLAB Function4/3(leakage)
  scalar to vector3/1(y) -> Integrator4/1
  Integrator4/1 -> Sum/2  "Coolant mass per node (kg)"
  Constant1/1 -> MinMax1/1, MATLAB Function18/3(M_total), Sum/1
  MATLAB Function7/1(y) -> Logical Operator/1
  Memory/1 -> Logical Operator/2
  Logical Operator/1 -> Detect Rise Positive/1, Memory/1
  Detect Rise Positive/1 -> MATLAB Function8/1(input)
  MATLAB Function10/1(Tin_c) -> MATLAB Function3/4(Tin_c), MATLAB Function12/4(Tinput_c), MATLAB Function15/2(Tinput_c), Tin_c/1  "Tin_c"
  MATLAB Function9/1(Tin_f) -> MATLAB Function3/5(Tin_f), MATLAB Function16/2(Tin_f), MATLAB Function5/7(Tin_f)
  MinMax1/1 -> MATLAB Function12/6(M_c), Out1/1, MATLAB Function18/2(M_actual)  "Coolant mass (kg)"
  Constant2/1 -> MATLAB Function19/1(h_wc)
  MATLAB Function19/1(h_wc_out) -> h_wc_out/1, MATLAB Function12/7(h_wc), MATLAB Function11/4(h_wc)
  Sum/1 -> MinMax1/2  "Coolant mass (kg)"
  MATLAB Function8/1(firstTrueTime) -> MATLAB Function4/4(check)
  MATLAB Function20/1(SG_fail) -> MATLAB Function10/3(SG_fail)
  Clock/1 -> MATLAB Function8/2(time), MATLAB Function10/5(t), MATLAB Function20/1(t), MATLAB Function4/1(time)
  MSLB/1 -> MATLAB Function20/3(MSLB)  "MSLB_time [s]"
  MSLB1/1 -> Product/1  "PDP1_fail"
  Product/1 -> MATLAB Function20/2(PDP_fail)
  MSLB2/1 -> Product/2  "PDP2_fail"

== matlab function SMDFR_lib/SMDFR/SMDFR/SMDFR 1/MATLAB Function4 ==
  data: time input; y output; LOCA_time input; leakage input; check input
function y = fcn(time,LOCA_time,leakage, check)

%add "&& check == 0" to the if to add the condition to stop the leakage
%once the reactor is failed
if time>=LOCA_time
    y = min(-1,-leakage*6+(time-LOCA_time)^(1/4)*leakage*1.1);
else
    y=0;
end

== matlab function SMDFR_lib/SMDFR/SMDFR/SMDFR 1/scalar to vector3 ==
  data: u input; y output size=1,3
function y = fcn(u)
y = zeros(1,3);
for i =1:3
    if i == 2
        y(i) = u*0.946;
    else
        y(i) = u*0.027;
    end
end

== matlab function SMDFR_lib/SMDFR/SMDFR/SMDFR 1/MATLAB Function5 ==
  data: Pi input size=3,1; dT_fdt output size=3,1; Te_f input size=3,1; T_f input size=3,1; T_w input size=3,1; c_pf parameter size=1,3; h_fw parameter size=1,3; A_fw parameter size=1,3; mdot_f input size=1,3; M_f input size=1,3; Tin_f input
function dT_fdt = eqn8(Pi, Te_f, T_f, T_w, c_pf, h_fw, A_fw, mdot_f, M_f, Tin_f)
dT_fdt=zeros(3,1);
for i = 1:3
    if i == 1
        dT_fdt(i) = ( Pi(i) + mdot_f(1) * c_pf(1) * (Tin_f - Te_f(1)) - h_fw(1)*A_fw(1)*(T_f(i) - T_w(i)) ) / (M_f(1) * c_pf(1));
    else
        dT_fdt(i) = ( Pi(i) + mdot_f(i) * c_pf(i) * (Te_f(i-1) - Te_f(i)) - h_fw(i)*A_fw(i)*(T_f(i) - T_w(i)) ) / (M_f(i) * c_pf(i));
    end
end

== matlab function SMDFR_lib/SMDFR/SMDFR/SMDFR 1/MATLAB Function7 ==
  data: u input; y output; fail_threshold parameter
function y = fcn(u,fail_threshold)

if max(u)>fail_threshold
    y=1;
else
    y=0;
end

== matlab function SMDFR_lib/SMDFR/SMDFR/SMDFR 1/MATLAB Function8 ==
  settings: updateMethod=DISCRETE
  data: input input; firstTrueTime output; time input
function firstTrueTime = f(input,time)
    persistent timeCaptured;
    persistent firstTime;
    if isempty(timeCaptured)
        timeCaptured = false;
        firstTime=0;
    end
    if input == 1 && ~timeCaptured
        firstTime = time;
        timeCaptured = true;
    end
    firstTrueTime = firstTime;
end

== matlab function SMDFR_lib/SMDFR/SMDFR/SMDFR 1/MATLAB Function11 ==
  data: T_f input size=3,1; T_w input size=3,1; dT_wdt output size=3,1; T_c input size=3,1; A_wc parameter size=1,3; A_fw parameter size=1,3; M_w parameter size=1,3; c_pw parameter size=1,3; h_wc input size=1,3; h_fw parameter size=1,3
function dT_wdt = eqn9(T_f, T_w, T_c, A_wc, A_fw, M_w, c_pw, h_wc, h_fw)
dT_wdt = zeros(3,1);
for i = 1:3
   dT_wdt(i) = ( h_fw(i)*A_fw(i)*(T_f(i) - T_w(i)) - h_wc(i)*A_wc(i)*(T_w(i) -T_c(i)) ) / (M_w(i) * c_pw(i));
end

== matlab function SMDFR_lib/SMDFR/SMDFR/SMDFR 1/MATLAB Function12 ==
  data: T_w input size=3,1; T_c input size=3,1; A_wc parameter size=1,3; dT_cdt output size=3,1; c_pc parameter size=1,3; Te_c input size=3,1; Tinput_c input; mdot_c input size=1,3; M_c input size=1,3; h_wc input size=1,3
function dT_cdt = eqn10(T_w, T_c, A_wc, c_pc, Te_c, Tinput_c, mdot_c, M_c, h_wc)
dT_cdt = zeros(3,1);
Tinput_c=Tinput_c(1);
for i = 1:3
    if i == 1
        dT_cdt(i) = ( mdot_c(i)*c_pc(i)*(Tinput_c - Te_c(i)) + h_wc(i)*A_wc(i)*(T_w(i) - T_c(i)) ) / (M_c(i) * c_pc(i));
    else
        dT_cdt(i) = ( mdot_c(i)*c_pc(i)*(Te_c(i-1) - Te_c(i)) + h_wc(i)*A_wc(i)*(T_w(i) - T_c(i)) ) / (M_c(i) * c_pc(i));
    end
end

== matlab function SMDFR_lib/SMDFR/SMDFR/SMDFR 1/MATLAB Function13 ==
  data: P output; N input; N_0 parameter; P_0 parameter
function P = eqn14(N, N_0, P_0)
%P = P_0;

P = (P_0/N_0) * N;

== matlab function SMDFR_lib/SMDFR/SMDFR/SMDFR 1/MATLAB Function14 ==
  data: Pi output size=3,1; P input; Pi_0 parameter size=1,3; P_0 parameter
function Pi = distr(P, Pi_0, P_0)
Pi = zeros(3,1);
%Pi = P_0*Pi_0';

for i = 1:3
    Pi(i) = P*Pi_0(i);
end

== matlab function SMDFR_lib/SMDFR/SMDFR/SMDFR 1/MATLAB Function15 ==
  data: T_c input size=3,1; Te_c output size=3,1; Tinput_c input; Tin_c parameter; Tout_c parameter
function Te_c  = cons1(T_c, Tinput_c, Tin_c, Tout_c)
%Te_c = tc_last;
Te_c = zeros(3,1); 
Te_c(2) = Tin_c;
Te_c(3) = Tout_c;
Te_c(1) = Tin_c;
for i = 1:3
    if i == 1
        Te_c(i) = 2*T_c(i) - Tinput_c;
    else
        Te_c(i) = 2*T_c(i) - Te_c(i-1);
    end
end

== matlab function SMDFR_lib/SMDFR/SMDFR/SMDFR 1/MATLAB Function16 ==
  data: T_f input size=3,1; Te_f output size=3,1; Tbar_f0 parameter; Tout_f parameter; Tin_f input
function Te_f = cons1(T_f, Tbar_f0, Tout_f, Tin_f)
%Te_f = tf_last;
Te_f = zeros(3,1);
Te_f(2) = Tin_f;
Te_f(3) = Tout_f;
Te_f(1) = Tin_f;
for i = 1:3
    if i == 1
        Te_f(i) = 2*T_f(i) - Tin_f;
    else
        Te_f(i) = 2*T_f(i) - Te_f(i-1);
    end
end

== matlab function SMDFR_lib/SMDFR/SMDFR/SMDFR 1/MATLAB Function17 ==
  data: Pi input size=3,1; sum_P output
function sum_P = fcn(Pi)

sum_P = sum(Pi);

== matlab function SMDFR_lib/SMDFR/SMDFR/SMDFR 1/MATLAB Function18 ==
  data: mdot_c input; y output; M_actual input; M_total input
function y = fcn(mdot_c,M_actual,M_total)
y=zeros(1,3);
for i=1:3
    %y(i) = mdot_c(i)+Auxiliary_leakage(i)*(time-LOCA_time);
    y(i) = mdot_c(i)*M_actual(i)/M_total(i);
end

== matlab function SMDFR_lib/SMDFR/SMDFR/SMDFR 1/MATLAB Function9 ==
  data: Tin_f output; Tf input
function Tin_f = fcn(Tf)

T_fo = Tf(end);
Tin_f=T_fo;

== matlab function SMDFR_lib/SMDFR/SMDFR/SMDFR 1/MATLAB Function19 ==
  data: h_wc input; h_wc_out output; mdot_c input
function h_wc_out = fcn(h_wc,mdot_c)

h_wc_out=zeros(1,3);
for i=1:3
    h_wc_out(i)=h_wc(i)*(mdot_c(i)/5550)^(0.8);
end

== matlab function SMDFR_lib/SMDFR/SMDFR/SMDFR 1/MATLAB Function20 ==
  data: t input; SG_fail output; PDP_fail input; MSLB input
function SG_fail = fcn(t,PDP_fail, MSLB)

t_empty = 40;

if t>(MSLB+t_empty) && PDP_fail==1
    SG_fail=1;
else
    SG_fail=0;
end

== matlab function SMDFR_lib/SMDFR/SMDFR/SMDFR 1/scalar to vector2 ==
  data: u input; y output size=1,3
function y = fcn(u)
y = zeros(1,3);
for i =1:3
    y(i) = u;
end

== matlab function SMDFR_lib/SMDFR/SMDFR/SMDFR 1/MATLAB Function6 ==
  data: u input; y output
function y = fcn(u)

y = mean(u);

== matlab function SMDFR_lib/Rankine/MATLAB Function ==
  data: T_in input; P output; p_in input; m_dot input; eta input
function P = Rankine(T_in,p_in,m_dot, eta)

%TURBINES

eta_t = 0.9;

%high pressure turbine inlet
Tht_in = T_in;
pht_in = p_in;
hht_in = XSteam('h_pT',pht_in,Tht_in);
Sht_in = XSteam('S_pT',pht_in,Tht_in);

%high pressure turbine bleed to heat exchanger
pht_bleed = 7;
%first IDEAL
Sht_bleed_id = Sht_in;
hht_bleed_id = XSteam('h_pS',pht_bleed,Sht_bleed_id);
%now REAL
hht_bleed = hht_in + (hht_bleed_id - hht_in) * eta_t;

%high pressure turbine outlet
pht_out = 1;
%first IDEAL
Sht_out_id = Sht_in;
hht_out_id = XSteam('h_pS',pht_out,Sht_out_id);
%now REAL
hht_out = hht_in + (hht_out_id - hht_in) * eta_t;

%low pressure turbine inlet
Tlt_in = 440;
plt_in = pht_out;
hlt_in = XSteam('h_pT',plt_in,Tlt_in);

%inlet

pcp_out = 3;
eta_p = 0.9;
%OPEN HEAT EXCHANGER (fluids in direct contact)

%the heat exchange is performed by the bleed STEAM from low pressure pump and the
%LIQUID from condenser

%inlet
poh_in = pcp_out;

%we can assume that the outlet is saturated liquid
poh_out = poh_in;
hoh_out = XSteam('hL_p',poh_out);
Soh_out = XSteam('SL_p',poh_out);

%HEAT EXCHANGER PUMP

%inlet
hhp_in = hoh_out;
Shp_in = Soh_out;

%the outlet pressure is the one of the SG inlet
php_out = p_in;
pch_in = php_out;

%first IDEAL
Shp_out_id = Shp_in;
hhp_out_id = XSteam('h_pS',php_out, Shp_out_id);

%now REAL
hhp_out = hhp_in + (hhp_out_id - hhp_in)/eta_p;

%CLOSED HEAT EXCHANGER (no contact between fluids)

%i assume that the steam bleed outlet is saturated liquid 
hchs_out = XSteam('hL_p',pht_bleed);

%outlet that goes to the SG 
pch_out = pch_in;
Tch_out = 205; %known
hch_out = XSteam('h_pT',pch_out,Tch_out);

%now i need bleed fractions for the mass flow rate
%from energy balance in the closed heat exchanger
y1 = abs((hch_out-hhp_out)/(hchs_out-hht_bleed));

Q = (hht_in - hch_out)*m_dot + (hlt_in - hht_out)*m_dot*(1-y1);

P=Q*eta;

== matlab function SMDFR_lib/Cu-Cl Cycle/Cu-Cl Cycle/Hydrolysis/MATLAB Function ==
  data: dT_hpdt output; V_hst input; d_hst input; C_hst input; G_hst input; h_hpi input; h_hpo input; K_h input; A_h input; T_hpo input; T_hpi input; T_hso input; T_hsi input
function dT_hpdt = CuCl_eqn1(V_hst,d_hst,C_hst,G_hst,h_hpi,h_hpo,K_h,A_h,T_hpo,T_hpi,T_hso,T_hsi)

dT_hpdt = G_hst/(V_hst*d_hst*C_hst)*(h_hpi-h_hpo)-K_h*A_h/(V_hst*d_hst*C_hst)*((T_hpo-T_hsi-T_hpi+T_hso)/log((T_hpo-T_hsi)/(T_hpi-T_hso)));

== matlab function SMDFR_lib/Cu-Cl Cycle/Cu-Cl Cycle/Hydrolysis/MATLAB Function1 ==
  data: dT_hsdt output; A_h20 input; A_cucl input; A_hcl input; A_cuocl input; M_h20 input; M_cucl input; M_hcl input; M_cuocl input; C_h20 input; C_cucl input; C_hcl input; C_cuocl input; K_h input; A_h input; T_hpo input; T_hsi input; T_hso input; T_hpi input; G_h20i input; G_h20o input; G_cucl input; G_hcl input; h_in input; h_out input; P_hydro input
function dT_hsdt = CuCl_eqn2(A_h20,A_cucl,A_hcl,A_cuocl,M_h20,M_cucl,M_hcl,M_cuocl,C_h20,C_cucl,C_hcl,C_cuocl,K_h,A_h,T_hpo,T_hsi,T_hso,T_hpi,G_h20i,G_h20o,G_cucl,G_hcl,h_in,h_out,P_hydro)

div = (A_h20*M_h20*C_h20+A_cucl*M_cucl*C_cucl+A_hcl*M_hcl*C_hcl+A_cuocl*M_cuocl*C_cuocl);

dT_hsdt = K_h*A_h*((T_hpo-T_hsi-T_hpi+T_hso)/log((T_hpo-T_hsi)/(T_hpi-T_hso)))/div+(G_cucl*C_cucl*T_hsi+G_h20i*h_in)/div-(G_hcl*C_hcl*T_hso+G_h20o*h_out)/div-P_hydro;

== matlab function SMDFR_lib/SMDFR/SMDFR/SMDFR 1/MATLAB Function1 ==
  data: Ce_i input size=6,1; dCei_dt output size=6,1; C_i input size=6,1; lambda_i parameter size=1,6; lambda_e parameter; lambda_c parameter; L parameter
function dCei_dt = eqn3(Ce_i, C_i, lambda_i, lambda_e, lambda_c, L)
dCei_dt = zeros(6,1); %!!!

for i=1:L 
    dCei_dt(i) = -lambda_i(i)*Ce_i(i) - lambda_e*Ce_i(i) + lambda_c*C_i(i) ;
end

== matlab function SMDFR_lib/Cu-Cl Cycle/Cu-Cl Cycle/Hydrolysis/MATLAB Function2 ==
  data: G_h20i input; G_h20o input; dN_h20dt output; v_h20 input
function dN_h20dt = CuCl_eqn3(G_h20i,G_h20o,v_h20)


dN_h20dt = G_h20i-G_h20o-v_h20;

== matlab function SMDFR_lib/Cu-Cl Cycle/Cu-Cl Cycle/Hydrolysis/MATLAB Function3 ==
  data: k_h input; v_h20 output; E_h input; T_hso input; M_hcl input; V_h input; p_h20 input
function v_h20 = CuCl_eqn4(k_h,E_h,T_hso,M_hcl,V_h,p_h20)

R = 8.31;
N = 1971.25;
p_hcl = M_hcl/V_h*R*T_hso;
v_h20 = k_h*exp(-E_h/(R*T_hso))*p_h20/p_hcl*N;
%v_h20 = 3;

== matlab function SMDFR_lib/Cu-Cl Cycle/Cu-Cl Cycle/Hydrolysis/MATLAB Function4 ==
  data: G_hcl input; v_h20 input; A_hcl input; dN_hcldt output; A_h20 input
function dN_hcldt = CuCl_eqn5(G_hcl,v_h20,A_hcl,A_h20)

v_hcl = 2*A_hcl*v_h20/A_h20;

dN_hcldt = v_hcl-G_hcl;

== matlab function SMDFR_lib/Cu-Cl Cycle/Cu-Cl Cycle/Hydrolysis/MATLAB Function5 ==
  data: G_cucl input; v_h20 input; A_cucl input; dN_cucldt output; A_h20 input
function dN_cucldt = CuCl_eqn6(G_cucl,v_h20,A_cucl,A_h20)

v_cucl = 2*A_cucl*v_h20/A_h20;

dN_cucldt = G_cucl-v_cucl;

== matlab function SMDFR_lib/Cu-Cl Cycle/Cu-Cl Cycle/Hydrolysis/MATLAB Function6 ==
  data: G_cuocl input; v_h20 input; A_cuocl input; dN_cuocldt output; A_h20 input
function dN_cuocldt = CuCl_eqn7(G_cuocl,v_h20,A_cuocl,A_h20)

v_cuocl = A_cuocl*v_h20/A_h20;

dN_cuocldt = v_cuocl-G_cuocl;

== matlab function SMDFR_lib/Cu-Cl Cycle/Cu-Cl Cycle/Decomposition/MATLAB Function ==
  data: V_dst input; dT_dpdt output; d_dst input; C_dst input; G_dst input; h_dpi input; h_dpo input; K_d input; A_d input; T_dpo input; T_dpi input; T_dso input; T_dsi input
function dT_dpdt = eqn1(V_dst,d_dst,C_dst,G_dst,h_dpi,h_dpo,K_d,A_d,T_dpo,T_dpi,T_dso,T_dsi)
div = V_dst*d_dst*C_dst;
dT_dpdt = G_dst/div*(h_dpi-h_dpo)-K_d*A_d/div*((T_dpo-T_dsi-T_dpi+T_dso)/log((T_dpo-T_dsi)/(T_dpi-T_dso)));

== matlab function SMDFR_lib/Cu-Cl Cycle/Cu-Cl Cycle/Decomposition/MATLAB Function1 ==
  data: A_cuocl input; dT_dsdt output; C_cuocl input; M_cuocl input; A_cucl input; C_cucl input; M_cucl input; A_o input; C_o input; M_o input; K_d input; A_d input; G_cuocl input; G_cucl input; G_o input; T_dpo input; T_dpi input; T_dso input; T_dsi input; P_decomposition input
function dT_dsdt = eqn2(A_cuocl,C_cuocl,M_cuocl,A_cucl,C_cucl,M_cucl,A_o,C_o,M_o,K_d,A_d,G_cuocl,G_cucl,G_o,T_dpo,T_dpi,T_dso,T_dsi,P_decomposition)
div = A_cuocl*C_cuocl*M_cuocl+A_cucl*C_cucl*M_cucl+A_o*C_o*M_o;
dT_dsdt = K_d*A_d/div*((T_dpo-T_dsi-T_dpi+T_dso)/log((T_dpo-T_dsi)/(T_dpi-T_dso)))+G_cuocl*C_cuocl*T_dsi-(G_cucl*C_cucl+G_o*C_o)*T_dso-P_decomposition;

== matlab function SMDFR_lib/Cu-Cl Cycle/Cu-Cl Cycle/Decomposition/MATLAB Function2 ==
  data: dM_cuocldt output; G_cuocl input; v_cuocl input
function dM_cuocldt = eqn3(G_cuocl,v_cuocl)

dM_cuocldt = G_cuocl-v_cuocl;

== matlab function SMDFR_lib/Cu-Cl Cycle/Cu-Cl Cycle/Decomposition/MATLAB Function3 ==
  data: v_cuocl output; A_cuocl input; k_d input; E_d input; T_dso input; M_o input; A_o input; V_d input
function v_cuocl = eqn4(A_cuocl,k_d,E_d,T_dso,M_o,A_o,V_d)
R = 8.31;
p_o = M_o*R*T_dso/(A_o*V_d);
v_cuocl = A_cuocl*k_d*exp(-E_d/(R*T_dso))/p_o;
v_cuocl = 35.63;

== matlab function SMDFR_lib/SMDFR/SMDFR/SMDFR 1/MATLAB Function ==
  data: N input; dC_idt output size=6,1; C_i input size=6,1; Ce_i input size=6,1; Lambda parameter; lambda_i parameter size=1,6; lambda_c parameter; lambda_e parameter; beta_i parameter size=1,6
function dC_idt = eqn2(N, C_i, Ce_i, Lambda, lambda_i, lambda_c, lambda_e, beta_i)
dC_idt = zeros(6,1);

for i=1:6
    dC_idt(i) = beta_i(i)/Lambda * N - lambda_i(i)*C_i(i) - lambda_c*C_i(i) + lambda_e*Ce_i(i);
end

== matlab function SMDFR_lib/Cu-Cl Cycle/Cu-Cl Cycle/Decomposition/MATLAB Function4 ==
  data: dM_cucldt output; G_cucl input; v_cuocl input; A_cucl input; A_cuocl input
function dM_cucldt = eqn5(G_cucl,v_cuocl,A_cucl,A_cuocl)
v_cucl = 2*A_cucl*v_cuocl/A_cuocl;
dM_cucldt = -G_cucl+v_cucl;

== matlab function SMDFR_lib/Cu-Cl Cycle/Cu-Cl Cycle/Decomposition/MATLAB Function5 ==
  data: dM_odt output; G_o input; v_cuocl input; A_o input; A_cuocl input
function dM_odt = eqn5(G_o,v_cuocl,A_o,A_cuocl)
v_o = A_o*v_cuocl/2/A_cuocl;
dM_odt = -G_o+v_o;

== matlab function SMDFR_lib/Cu-Cl Cycle/Cu-Cl Cycle/Electrolysis/MATLAB Function ==
  data: v_h2 input; dN_cucl2dt output; G_cucl2 input; A_cucl2 input; A_h2 input
function dN_cucl2dt = eqn1(v_h2,G_cucl2,A_cucl2,A_h2)
v_cucl = 2*v_h2*A_cucl2/A_h2*1.05;
dN_cucl2dt = v_cucl - G_cucl2;

== matlab function SMDFR_lib/Cu-Cl Cycle/Cu-Cl Cycle/Electrolysis/MATLAB Function1 ==
  data: v_h2 input; dN_cucldt output; G_cucl input; A_cucl input; A_h2 input
function dN_cucldt = eqn2(v_h2,G_cucl,A_cucl,A_h2)
v_cucl = 2*v_h2*A_cucl/A_h2;
dN_cucldt = -v_cucl + G_cucl;

== matlab function SMDFR_lib/Cu-Cl Cycle/Cu-Cl Cycle/Electrolysis/MATLAB Function2 ==
  data: v_h2 input; dN_h2dt output; G_h2 input
function dN_h2dt = eqn3(v_h2,G_h2)

dN_h2dt = v_h2 - G_h2;

== matlab function SMDFR_lib/Cu-Cl Cycle/Cu-Cl Cycle/Electrolysis/MATLAB Function3 ==
  data: v_h2 input; dN_hcldt output; G_hcl input; A_hcl input; A_h2 input
function dN_hcldt = eqn4(v_h2,G_hcl,A_hcl,A_h2)
v_hcl = 2*v_h2*A_hcl/A_h2;
dN_hcldt = -v_hcl + G_hcl;

== matlab function SMDFR_lib/Cu-Cl Cycle/Cu-Cl Cycle/Electrolysis/MATLAB Function4 ==
  data: k_e input; v_h2 output; E_e input; T_es input; M_hcl input; M_cucl input; M_hcl0 input; M_cucl0 input; p_h20 input; M_h2 input; A_h2 input; V_h2 input; M_cucl20 input; M_cucl2 input
function v_h2 = eqn5(k_e,E_e,T_es,M_hcl,M_cucl,M_hcl0,M_cucl0,p_h20,M_h2,A_h2,V_h2,M_cucl20,M_cucl2)
R = 8.31;
p_h2 = M_h2/(A_h2*V_h2)*R*T_es;
v_h2 = k_e*exp(-E_e/(R*T_es))*(M_hcl*M_cucl/(M_hcl0*M_cucl0))*(M_cucl20/M_cucl2)*(p_h2/p_h20)^(-0.5);

== matlab function SMDFR_lib/HTE/HTE/MATLAB Function ==
  data: k_hte input; v_h20 output; E_hte input; T_hte input; M_h2 input; A_h2 input; V_c input; p_h20 input
function v_h20 = eqn1(k_hte,E_hte,T_hte,M_h2,A_h2,V_c,p_h20)

R = 8.31;
p_h2 = M_h2*R*T_hte/A_h2/V_c;
v_h20 = k_hte*exp(-E_hte/R/T_hte)*p_h20/p_h2;

== matlab function SMDFR_lib/HTE/HTE/MATLAB Function1 ==
  data: G_h20 input; dN_h20dt output; G_h20o input; v_h20 input; A_h20 input
function dN_h20dt = eqn2(G_h20,G_h20o,v_h20,A_h20)
v_h20 = v_h20*A_h20;
dN_h20dt = G_h20-G_h20o-v_h20;

== matlab function SMDFR_lib/ACS/ACS_fun ==
  data: state input; GA output; ACS_flow input; time input; LOCA_time input; ACS_response_time input; SG_time input
function GA  = ACS(state,ACS_flow,time,LOCA_time,ACS_response_time, SG_time)

if state && ((time-LOCA_time) > ACS_response_time || (time-SG_time) > ACS_response_time)
    GA = ACS_flow;
else
    GA = 0;
end

== matlab function SMDFR_lib/HTE/HTE/MATLAB Function3 ==
  data: G_h2 input; dN_h2dt output; v_h20 input; A_h2 input
function dN_h2dt = eqn3(G_h2,v_h20,A_h2)
v_h2 = v_h20*A_h2;
dN_h2dt = -G_h2+v_h2;

== matlab function SMDFR_lib/SMDFR/SMDFR/SMDFR 1/MATLAB Function2 ==
  data: rho input; dN_dt output; N input; C_i input size=6,1; lambda_i parameter size=1,6; beta parameter; Lambda parameter; L parameter
function dN_dt = eqn4(rho, N, C_i, lambda_i, beta, Lambda, L)
sum_i = 0;

for i=1:L 
    sum_i = sum_i + lambda_i(i)*C_i(i);
end

dN_dt = (rho - beta)*(N/Lambda) + sum_i;

== matlab function SMDFR_lib/SMDFR/SMDFR/SMDFR 1/MATLAB Function3 ==
  data: rho_ext input; rho output; rho_0 parameter; Te_f input size=3,1; Te_c input size=3,1; Tbar_f0 parameter; Tbar_c0 parameter; alfa_f parameter; alfa_c parameter; Tin_c input; Tin_f input
function rho = eqn15(rho_ext, rho_0, Te_f, Te_c, Tbar_f0, Tbar_c0, alfa_f, alfa_c, Tin_c, Tin_f)

rho = rho_0 + alfa_f*(mean([Te_f(3),Tin_f]) - Tbar_f0) + alfa_c*(mean([Te_c(3),Tin_c]) - Tbar_c0) + rho_ext;

== matlab function SMDFR_lib/SMDFR/SMDFR/SMDFR 1/Average ==
  data: u input; y output
function y = fcn(u)

y = mean(u);

== matlab function SMDFR_lib/SMDFR/SMDFR/SMDFR 1/MATLAB Function10 ==
  settings: updateMethod=DISCRETE
  data: Tc input; Tin_c output; C_c parameter; mdot_c input; SG_fail input; m_dot_ACS input; t input
function Tin_c = fcn(Tc, C_c, mdot_c, SG_fail, m_dot_ACS, t)

persistent first_SG_fail_time

% Initialize first_SG_fail_time to -1 if it hasn't been initialized yet
if isempty(first_SG_fail_time)
    first_SG_fail_time = -1;
end

Tout_c = Tc(end);
Q = 8.2564e+07 * 1.85 * 3.64;
Q = Q * mdot_c(1) / 5550 / 2 - (5500 - mdot_c(1));
Tin = 973;

if SG_fail
    if first_SG_fail_time == -1
        first_SG_fail_time = t; % Store the first time SG_fail is 1
    end
    Q = max(0, Q + Q * (first_SG_fail_time - t) / (300));
    Tin = 873;
else
    if first_SG_fail_time ~= -1
        first_SG_fail_time = -1; % Reset the first_SG_fail_time to -1 when SG_fail becomes 0
    end
end

Tin_c_temp = Tout_c - Q / (sum(mdot_c) * C_c);
Tin_c = Tin_c_temp * (sum(mdot_c) - m_dot_ACS) / sum(mdot_c) + Tin * m_dot_ACS / sum(mdot_c);
